simulink model "FCC_replacement"  (R2019b)
settings: Solver=FixedStepDiscrete  StartTime=0.0  StopTime=10.0  FixedStep=0.001  RelTol=1e-3  EnableMultiTasking=on
undefined symbols (not defined in the file or in its folder): DiscIntNeverNeededParam
libraries: simulink x10, HeliLibrary x3
Description:
  | This model represents a flight control system for a helicopter that controls pitch attitude, roll attitude and yaw rate based on pilot inputs from the cyclic and pedals. The flight control computer also closes the loop on three hydrualic actuators and has sensor inputs from three Attitude/Heading Reference Systems.
settings Model: DataDictionary=HeliSystemDD.sldd  sldv_blockreplacement_configurable_lib=FCC_rt_lib  Creator=bpotter  LastModifiedBy=bpotter
settings DataIOCC: LimitDataPoints=on  ReturnWorkspaceOutputs=off
settings OptimizationCC: BlockReduction=off  DefaultParameterBehavior=Inlined  UseDivisionForNetSlopeComputation=on  InitFltsAndDblsToZero=on  EfficientFloat2IntCast=on  EfficientMapNaN2IntZero=off  LifeSpan=inf  MaxStackSize=inf  EfficientTunableParamExpr=on
settings DebuggingCC: SignalInfNanChecking=error  SignalRangeChecking=error  ReadBeforeWriteMsg=EnableAllAsError  WriteAfterWriteMsg=EnableAllAsError  WriteAfterReadMsg=EnableAllAsError  AlgebraicLoopMsg=error  ArtificialAlgebraicLoopMsg=error  SaveWithDisabledLinksMsg=error  SaveWithParameterizedLinksMsg=none  BlockPriorityViolationMsg=error  SolverPrmCheckMsg=error  InheritedTsInSrcMsg=error  SingleTaskRateTransMsg=error  TasksWithSamePriorityMsg=error  SigSpecEnsureSampleTimeMsg=error  CheckMatrixSingularityMsg=error  IntegerOverflowMsg=error  ParameterUnderflowMsg=error  ParameterPrecisionLossMsg=error  ParameterTunabilityLossMsg=error  UnderSpecifiedDataTypeMsg=error  UnnecessaryDatatypeConvMsg=warning  VectorMatrixConversionMsg=error  UnconnectedInputMsg=error  UnconnectedOutputMsg=error  UnconnectedLineMsg=error  SFcnCompatibilityMsg=error  UniqueDataStoreMsg=warning  BusObjectLabelMismatch=error  RootOutportRequireBusObject=error  AssertControl=DisableAll  AllowSymbolicDim=off  ModelReferenceIOMsg=error  ModelReferenceIOMismatchMessage=error  UnknownTsInhSupMsg=error  ModelReferenceDataLoggingMessage=error  StateNameClashWarn=warning  PregeneratedLibrarySubsystemCodeDiagnostic=none  StrictBusMsg=ErrorOnBusTreatedAsVector  NonBusSignalsTreatedAsBus=error  SFInvalidInputDataAccessInChartInitDiag=error  SFTransitionOutsideNaturalParentDiag=error  SFUnreachableExecutionPathDiag=error  SFUndirectedBroadcastEventsDiag=error  SFTransitionActionBeforeConditionDiag=error  SFExecutionAtInitializationDiag=none  IntegerSaturationMsg=error  ArithmeticOperatorsInVariantConditions=warning
settings HardwareCC: ProdBitPerPointer=32  ProdBitPerSizeT=32  ProdBitPerPtrDiffT=32  ProdWordSize=32  ProdHWDeviceType=Intel->x86-32 (Windows32)  TargetIntDivRoundTo=Zero
settings ModelReferenceCC: ModelReferenceNumInstancesAllowed=Single  PropagateSignalLabelsOutOfModel=off
settings SFSimCC: SimUseLocalCustomCode=off  CompileTimeRecursionLimit=0  EnableRuntimeRecursion=off  MATLABDynamicMemAlloc=off  CustomCodeUndefinedFunction=UseInterfaceOnly
settings RTWCC: SystemTargetFile=ert.tlc  TemplateMakefile=ert_default_tmf  GenerateReport=on  RTWUseLocalCustomCode=off  IncludeHyperlinkInReport=on  LaunchReport=on  PortableWordSizes=on  GenerateTraceInfo=on  GenerateTraceReport=on  GenerateTraceReportSl=on  GenerateTraceReportSf=on  GenerateTraceReportEml=on
settings CodeAppCC: ForceParamTrailComments=on  IgnoreCustomStorageClasses=off  MATLABFcnDesc=on  MangleLength=4  StateflowObjectComments=on  ReqsInCode=on
settings ERTTargetCC: TargetLangStandard=C99 (ISO)  UtilityFuncGeneration=Shared location  MultiwordLength=2048  GenerateSampleERTMain=on  IncludeMdlTerminateFcn=off  SuppressErrorStatus=on  SupportAbsoluteTime=off  SupportNonFinite=off  ParenthesesLevel=Maximum  CastingMode=Standards  GenerateSharedConstants=off  ERTCustomFileTemplate=example_file_process.tlc  ERTFilePackagingFormat=Compact  PreserveExpressionOrder=on  PreserveIfCondition=on  ConvertIfToSwitch=off  SuppressUnreachableDefaultCases=off  EnableSignedLeftShifts=off  EnableSignedRightShifts=off
settings ConfigComp: CovMetricSettings=dw  CovHtmlReporting=on  CovSaveCumulativeToWorkspaceVar=on  CovSaveSingleToWorkspaceVar=on  CovExternalEMLEnable=off  CovSFcnEnable=off  DVTestSuiteOptimization=CombinedObjectives (Nonlinear Extended)  DVDetectOutOfBounds=on  DVDesignMinMaxCheck=on  DVRebuildModelRepresentation=Always

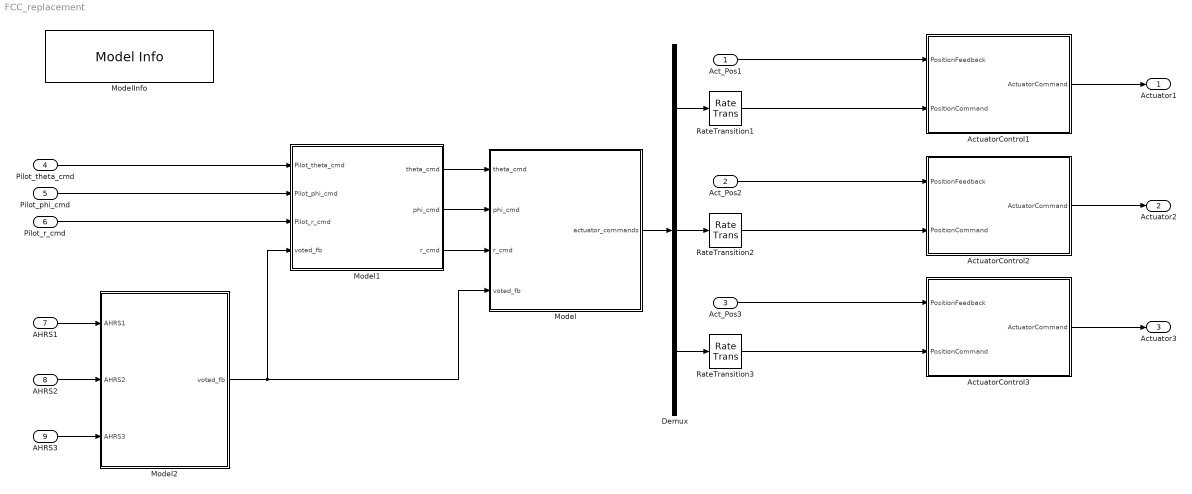
== system FCC_replacement ==
  Act_Pos1 : Inport  RequirementInfo={} %GIDa_bd07c6dd_f370_4b97_930d_e4b4981f6696  OutMin=-32768  OutMax=32767  OutDataTypeStr=int16  PortDimensions=1  SampleTime=0.001
  Act_Pos2 : Inport  RequirementInfo={} %GIDa_befe8f2a_df1a_408c_ad43_982e86d61679  Port=2  OutMin=-32768  OutMax=32767  OutDataTypeStr=int16  PortDimensions=1  SampleTime=0.001
  Act_Pos3 : Inport  RequirementInfo={} %GIDa_31a40888_6c46_41b4_95a0_85353469c339  Port=3  OutMin=-32768  OutMax=32767  OutDataTypeStr=int16  PortDimensions=1  SampleTime=0.001
  Pilot_theta_cmd : Inport  RequirementInfo={} %GIDa_db7610c8_fc0b_436a_9176_d063f912f7d4  Port=4  OutMin=-32768  OutMax=32767  OutDataTypeStr=int16  PortDimensions=1  SampleTime=0.01
  Pilot_phi_cmd : Inport  RequirementInfo={} %GIDa_c88793d4_8072_44c9_b7b8_fa9c7a9d095b  Port=5  OutMin=-32768  OutMax=32767  OutDataTypeStr=int16  PortDimensions=1  SampleTime=0.01
  Pilot_r_cmd : Inport  RequirementInfo={} %GIDa_dcbca35e_d37f_4666_ab6e_90461c32e72b  Port=6  OutMin=-32768  OutMax=32767  OutDataTypeStr=int16  PortDimensions=1  SampleTime=0.01
  AHRS1 : Inport  RequirementInfo={} %GIDa_80750aa2_e003_442f_b031_591405abb5b4  Port=7  OutDataTypeStr=Bus: AHRS_Bus  PortDimensions=1  SampleTime=0.01  BusOutputAsStruct=on
  AHRS2 : Inport  RequirementInfo={} %GIDa_426ecfe9_991d_4f5f_80a1_3ebd9c43cb2d  Port=8  OutDataTypeStr=Bus: AHRS_Bus  PortDimensions=1  SampleTime=0.01  BusOutputAsStruct=on
  AHRS3 : Inport  RequirementInfo={} %GIDa_78c653e8_6a57_498e_82a6_5c1330482b46  Port=9  OutDataTypeStr=Bus: AHRS_Bus  PortDimensions=1  SampleTime=0.01  BusOutputAsStruct=on
  ActuatorControl1 : Subsystem  TreatAsAtomicUnit=on  mask(Sldv ModelReference(Model name:ActuatorLoop) Replacement){ModelName=ActuatorLoop, ParameterArgumentNames=Kp,Kd,Ki, ParameterArgumentValuesAsString=0.00272,2.73,0.339, SimulationMode=Normal, Kd=0.00272, Ki=2.73, Kp=0.339}
      mask help: Replacement for the Model Reference block that references the model ActuatorLoop. If Model arguments are specified on the Model Reference block, then they will appear in the mask parameters.
  ActuatorControl2 : Subsystem  TreatAsAtomicUnit=on  mask(Sldv ModelReference(Model name:ActuatorLoop) Replacement){ModelName=ActuatorLoop, ParameterArgumentNames=Kp,Kd,Ki, ParameterArgumentValuesAsString=0.00272,2.73,0.339, SimulationMode=Normal, Kd=0.00272, Ki=2.73, Kp=0.339}
      mask help: Replacement for the Model Reference block that references the model ActuatorLoop. If Model arguments are specified on the Model Reference block, then they will appear in the mask parameters.
  ActuatorControl3 : Subsystem  TreatAsAtomicUnit=on  mask(Sldv ModelReference(Model name:ActuatorLoop) Replacement){ModelName=ActuatorLoop, ParameterArgumentNames=Kp,Kd,Ki, ParameterArgumentValuesAsString=0.00272,2.73,0.339, SimulationMode=Normal, Kd=0.00272, Ki=2.73, Kp=0.339}
      mask help: Replacement for the Model Reference block that references the model ActuatorLoop. If Model arguments are specified on the Model Reference block, then they will appear in the mask parameters.
  Demux : Demux  Outputs=3
  Model : Subsystem  TreatAsAtomicUnit=on  mask(Sldv ModelReference(Model name:Heli_inner_loop) Replacement){ModelName=Heli_inner_loop, ParameterArgumentNames=, ParameterArgumentValuesAsString=, SimulationMode=Normal}
      mask help: Replacement for the Model Reference block that references the model Heli_inner_loop. If Model arguments are specified on the Model Reference block, then they will appear in the mask parameters.
  Model1 : Subsystem  TreatAsAtomicUnit=on  mask(Sldv ModelReference(Model name:Heli_outer_loop) Replacement){ModelName=Heli_outer_loop, ParameterArgumentNames=, ParameterArgumentValuesAsString=, SimulationMode=Normal}
      mask help: Replacement for the Model Reference block that references the model Heli_outer_loop. If Model arguments are specified on the Model Reference block, then they will appear in the mask parameters.
  Model2 : Subsystem  TreatAsAtomicUnit=on  mask(Sldv ModelReference(Model name:AHRS_voter) Replacement){ModelName=AHRS_voter, ParameterArgumentNames=, ParameterArgumentValuesAsString=, SimulationMode=Normal}
      mask help: Replacement for the Model Reference block that references the model AHRS_voter. If Model arguments are specified on the Model Reference block, then they will appear in the mask parameters.
  ModelInfo : simulink/Model-Wide Utilities/Model Info  Frame=on  DisplayStringWithTags=|  HorizontalTextAlignment=Center  LeftAlignmentValue=0.5
      | Model Name: %<ModelName>
      | Model Version: %<ModelVersion>
      | Last Modified: %<LastModificationDate>
      | 
      | Copyright 2016 The MathWorks, Inc.
  RateTransition1 : RateTransition  OutPortSampleTime=0.001
  RateTransition2 : RateTransition  OutPortSampleTime=0.001
  RateTransition3 : RateTransition  OutPortSampleTime=0.001
  Actuator1 : Outport  RequirementInfo={} %GIDa_0e27a381_736b_4604_a443_1ce3b6bc89bb  VectorParamsAs1DForOutWhenUnconnected=off
  Actuator2 : Outport  RequirementInfo={} %GIDa_ad165c3e_4ab6_4671_aa0b_225d448592bb  Port=2  VectorParamsAs1DForOutWhenUnconnected=off
  Actuator3 : Outport  RequirementInfo={} %GIDa_f2f33165_edb5_46cb_9250_52960ae67539  Port=3  VectorParamsAs1DForOutWhenUnconnected=off
  wires:
  RateTransition1/1 -> ActuatorControl1/2(PositionCommand)
  RateTransition2/1 -> ActuatorControl2/2(PositionCommand)
  RateTransition3/1 -> ActuatorControl3/2(PositionCommand)
  AHRS2/1 -> Model2/2(AHRS2)
  AHRS3/1 -> Model2/3(AHRS3)
  Demux/1 -> RateTransition1/1
  Demux/2 -> RateTransition2/1
  Demux/3 -> RateTransition3/1
  Model/1(actuator_commands) -> Demux/1
  Model1/1(theta_cmd) -> Model/1(theta_cmd)
  Model1/2(phi_cmd) -> Model/2(phi_cmd)
  Model1/3(r_cmd) -> Model/3(r_cmd)
  AHRS1/1 -> Model2/1(AHRS1)
  Pilot_theta_cmd/1 -> Model1/1(Pilot_theta_cmd)
  Pilot_phi_cmd/1 -> Model1/2(Pilot_phi_cmd)
  Pilot_r_cmd/1 -> Model1/3(Pilot_r_cmd)
  Act_Pos1/1 -> ActuatorControl1/1(PositionFeedback)
  Act_Pos2/1 -> ActuatorControl2/1(PositionFeedback)
  Act_Pos3/1 -> ActuatorControl3/1(PositionFeedback)
  ActuatorControl1/1(ActuatorCommand) -> Actuator1/1
  ActuatorControl2/1(ActuatorCommand) -> Actuator2/1
  ActuatorControl3/1(ActuatorCommand) -> Actuator3/1
  Model2/1(voted_fb) -> Model/4(voted_fb), Model1/4(voted_fb)

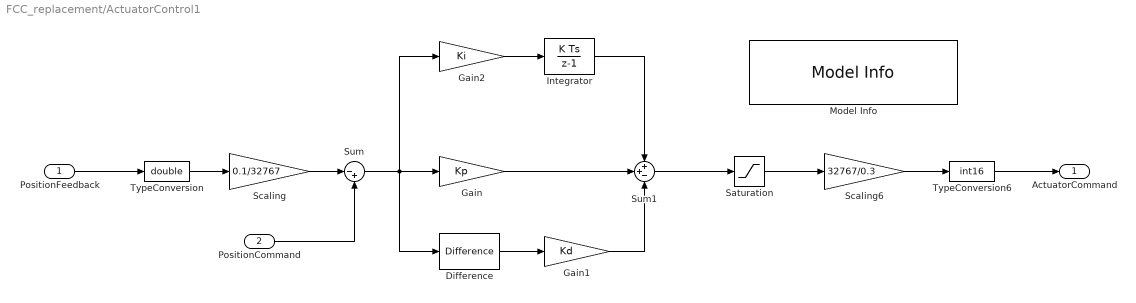
== system FCC_replacement/ActuatorControl1 ==
  PositionFeedback : Inport  OutMin=-32768  OutMax=32767  OutDataTypeStr=int16  PortDimensions=1  SampleTime=[0.001,0]
  PositionCommand : Inport  Port=2  OutMin=-0.1  OutMax=0.1  OutDataTypeStr=double  PortDimensions=1  SampleTime=[0.001,0]
  Difference : simulink/Discrete/Difference  ICPrevInput=0.0  OutMin=[]  OutMax=[]  OutDataType=fixdt(1, 16)  OutScaling=2^-10  DoSatur=off
  Gain : Gain  Gain=Kp
  Gain1 : Gain  Gain=Kd
  Gain2 : Gain  Gain=Ki
  Integrator : DiscreteIntegrator  SampleTime=-1  LimitOutput=on  UpperSaturationLimit=0.1  LowerSaturationLimit=-0.1  ICPrevOutput=DiscIntNeverNeededParam  ICPrevScaledInput=DiscIntNeverNeededParam
      settings: AttributesFormatString="%<LowerSaturationLimit> to  %<UpperSaturationLimit>"
  Model Info : simulink/Model-Wide Utilities/Model Info  Frame=on  DisplayStringWithTags=|  HorizontalTextAlignment=Center  LeftAlignmentValue=0.5
      | Model Name: %<ModelName>
      | Model Version: %<ModelVersion>
      | Last Modified: %<LastModificationDate>
      | 
      | Copyright 2016 The MathWorks, Inc.
  Saturation : Saturate  UpperLimit=0.3  LowerLimit=-0.3
      settings: AttributesFormatString=%<LowerLimit> to %<UpperLimit>
  Scaling : Gain  Gain=0.1/32767
  Scaling6 : Gain  Gain=32767/0.3  SaturateOnIntegerOverflow=on  OutDataTypeStr=Inherit: Same as input
  Sum : Sum  Inputs=|-+
  Sum1 : Sum  Inputs=++-
  TypeConversion : DataTypeConversion  OutDataTypeStr=double
  TypeConversion6 : DataTypeConversion  OutDataTypeStr=int16
  ActuatorCommand : Outport  OutDataTypeStr=int16  PortDimensions=1  SampleTime=[0.001,0]  VectorParamsAs1DForOutWhenUnconnected=off
  wires:
  TypeConversion6/1 -> ActuatorCommand/1
  Saturation/1 -> Scaling6/1
  Scaling6/1 -> TypeConversion6/1
  Scaling/1 -> Sum/1
  TypeConversion/1 -> Scaling/1
  PositionFeedback/1 -> TypeConversion/1
  Gain2/1 -> Integrator/1
  Gain1/1 -> Sum1/3
  Difference/1 -> Gain1/1
  Integrator/1 -> Sum1/1
  Sum1/1 -> Saturation/1
  Gain/1 -> Sum1/2
  Sum/1 -> Difference/1, Gain2/1, Gain/1
  PositionCommand/1 -> Sum/2

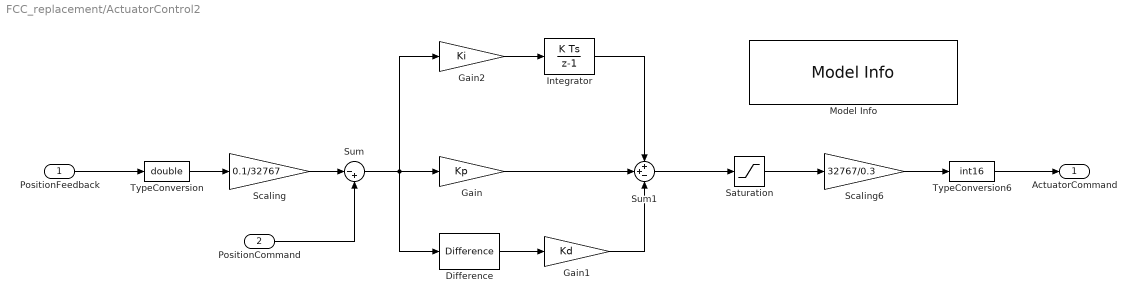
== system FCC_replacement/ActuatorControl2 ==
  PositionFeedback : Inport  OutMin=-32768  OutMax=32767  OutDataTypeStr=int16  PortDimensions=1  SampleTime=[0.001,0]
  PositionCommand : Inport  Port=2  OutMin=-0.1  OutMax=0.1  OutDataTypeStr=double  PortDimensions=1  SampleTime=[0.001,0]
  Difference : simulink/Discrete/Difference  ICPrevInput=0.0  OutMin=[]  OutMax=[]  OutDataType=fixdt(1, 16)  OutScaling=2^-10  DoSatur=off
  Gain : Gain  Gain=Kp
  Gain1 : Gain  Gain=Kd
  Gain2 : Gain  Gain=Ki
  Integrator : DiscreteIntegrator  SampleTime=-1  LimitOutput=on  UpperSaturationLimit=0.1  LowerSaturationLimit=-0.1  ICPrevOutput=DiscIntNeverNeededParam  ICPrevScaledInput=DiscIntNeverNeededParam
      settings: AttributesFormatString="%<LowerSaturationLimit> to  %<UpperSaturationLimit>"
  Model Info : simulink/Model-Wide Utilities/Model Info  Frame=on  DisplayStringWithTags=|  HorizontalTextAlignment=Center  LeftAlignmentValue=0.5
      | Model Name: %<ModelName>
      | Model Version: %<ModelVersion>
      | Last Modified: %<LastModificationDate>
      | 
      | Copyright 2016 The MathWorks, Inc.
  Saturation : Saturate  UpperLimit=0.3  LowerLimit=-0.3
      settings: AttributesFormatString=%<LowerLimit> to %<UpperLimit>
  Scaling : Gain  Gain=0.1/32767
  Scaling6 : Gain  Gain=32767/0.3  SaturateOnIntegerOverflow=on  OutDataTypeStr=Inherit: Same as input
  Sum : Sum  Inputs=|-+
  Sum1 : Sum  Inputs=++-
  TypeConversion : DataTypeConversion  OutDataTypeStr=double
  TypeConversion6 : DataTypeConversion  OutDataTypeStr=int16
  ActuatorCommand : Outport  OutDataTypeStr=int16  PortDimensions=1  SampleTime=[0.001,0]  VectorParamsAs1DForOutWhenUnconnected=off
  wires:
  TypeConversion6/1 -> ActuatorCommand/1
  Saturation/1 -> Scaling6/1
  Scaling6/1 -> TypeConversion6/1
  Scaling/1 -> Sum/1
  TypeConversion/1 -> Scaling/1
  PositionFeedback/1 -> TypeConversion/1
  Gain2/1 -> Integrator/1
  Gain1/1 -> Sum1/3
  Difference/1 -> Gain1/1
  Integrator/1 -> Sum1/1
  Sum1/1 -> Saturation/1
  Gain/1 -> Sum1/2
  Sum/1 -> Difference/1, Gain2/1, Gain/1
  PositionCommand/1 -> Sum/2

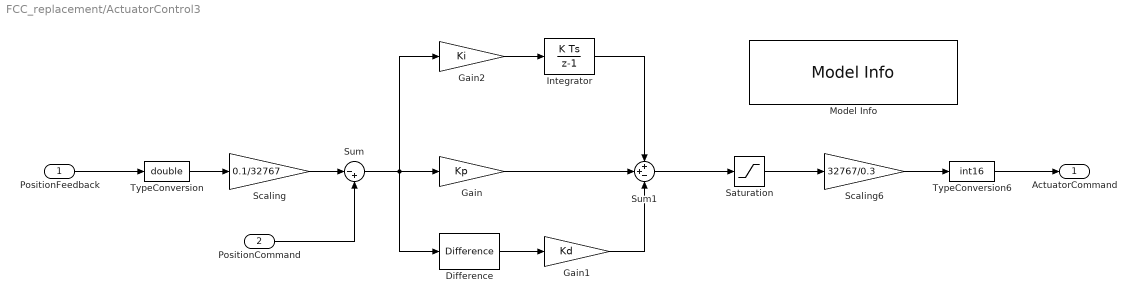
== system FCC_replacement/ActuatorControl3 ==
  PositionFeedback : Inport  OutMin=-32768  OutMax=32767  OutDataTypeStr=int16  PortDimensions=1  SampleTime=[0.001,0]
  PositionCommand : Inport  Port=2  OutMin=-0.1  OutMax=0.1  OutDataTypeStr=double  PortDimensions=1  SampleTime=[0.001,0]
  Difference : simulink/Discrete/Difference  ICPrevInput=0.0  OutMin=[]  OutMax=[]  OutDataType=fixdt(1, 16)  OutScaling=2^-10  DoSatur=off
  Gain : Gain  Gain=Kp
  Gain1 : Gain  Gain=Kd
  Gain2 : Gain  Gain=Ki
  Integrator : DiscreteIntegrator  SampleTime=-1  LimitOutput=on  UpperSaturationLimit=0.1  LowerSaturationLimit=-0.1  ICPrevOutput=DiscIntNeverNeededParam  ICPrevScaledInput=DiscIntNeverNeededParam
      settings: AttributesFormatString="%<LowerSaturationLimit> to  %<UpperSaturationLimit>"
  Model Info : simulink/Model-Wide Utilities/Model Info  Frame=on  DisplayStringWithTags=|  HorizontalTextAlignment=Center  LeftAlignmentValue=0.5
      | Model Name: %<ModelName>
      | Model Version: %<ModelVersion>
      | Last Modified: %<LastModificationDate>
      | 
      | Copyright 2016 The MathWorks, Inc.
  Saturation : Saturate  UpperLimit=0.3  LowerLimit=-0.3
      settings: AttributesFormatString=%<LowerLimit> to %<UpperLimit>
  Scaling : Gain  Gain=0.1/32767
  Scaling6 : Gain  Gain=32767/0.3  SaturateOnIntegerOverflow=on  OutDataTypeStr=Inherit: Same as input
  Sum : Sum  Inputs=|-+
  Sum1 : Sum  Inputs=++-
  TypeConversion : DataTypeConversion  OutDataTypeStr=double
  TypeConversion6 : DataTypeConversion  OutDataTypeStr=int16
  ActuatorCommand : Outport  OutDataTypeStr=int16  PortDimensions=1  SampleTime=[0.001,0]  VectorParamsAs1DForOutWhenUnconnected=off
  wires:
  TypeConversion6/1 -> ActuatorCommand/1
  Saturation/1 -> Scaling6/1
  Scaling6/1 -> TypeConversion6/1
  Scaling/1 -> Sum/1
  TypeConversion/1 -> Scaling/1
  PositionFeedback/1 -> TypeConversion/1
  Gain2/1 -> Integrator/1
  Gain1/1 -> Sum1/3
  Difference/1 -> Gain1/1
  Integrator/1 -> Sum1/1
  Sum1/1 -> Saturation/1
  Gain/1 -> Sum1/2
  Sum/1 -> Difference/1, Gain2/1, Gain/1
  PositionCommand/1 -> Sum/2

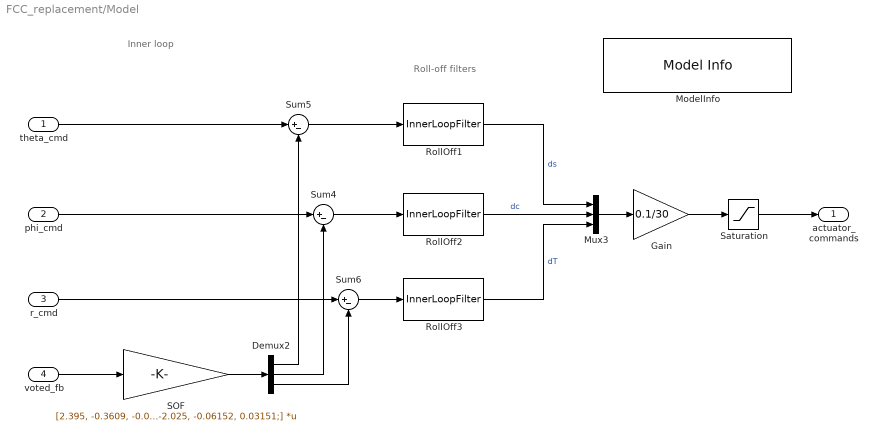
== system FCC_replacement/Model ==
  note: Inner loop
  note: Roll-off filters
  theta_cmd : Inport  OutMin=-30  OutMax=30  OutDataTypeStr=double  PortDimensions=1  SampleTime=[0.01,0]
  phi_cmd : Inport  Port=2  OutMin=-30  OutMax=30  OutDataTypeStr=double  PortDimensions=1  SampleTime=[0.01,0]
  r_cmd : Inport  Port=3  OutMin=-30  OutMax=30  OutDataTypeStr=double  PortDimensions=1  SampleTime=[0.01,0]
  voted_fb : Inport  Port=4  OutMin=-180  OutMax=180  OutDataTypeStr=double  PortDimensions=5  SampleTime=[0.01,0]
  Demux2 : Demux  Outputs=3
  Gain : Gain  Gain=0.1/30
  ModelInfo : simulink/Model-Wide Utilities/Model Info  Frame=on  DisplayStringWithTags=|  HorizontalTextAlignment=Center  LeftAlignmentValue=0.5
      | Model Name: %<ModelName>
      | Model Version: %<ModelVersion>
      | Last Modified: %<LastModificationDate>
      | 
      | Copyright 2016 The MathWorks, Inc.
  Mux3 : Mux  Inputs=3
  RollOff1 : HeliLibrary/InnerLoopFilter  Tag=FilterWizardSubSystem  SystemSampleTime=-1  Latency=0  AutoFrameSizeCalculation=off
      settings: AttributesFormatString=@100Hz
  RollOff2 : HeliLibrary/InnerLoopFilter  Tag=FilterWizardSubSystem  SystemSampleTime=-1  Latency=0  AutoFrameSizeCalculation=off
      settings: AttributesFormatString=@100Hz
  RollOff3 : HeliLibrary/InnerLoopFilter  Tag=FilterWizardSubSystem  SystemSampleTime=-1  Latency=0  AutoFrameSizeCalculation=off
      settings: AttributesFormatString=@100Hz
  SOF : Gain  Gain=[2.395, -0.3609, -0.002145, 0.8087, -0.0205; -0.1427, -1.115, 0.04573, -0.04318, -0.1007; -0.02792, -0.02229, -2.025, -0.06152, 0.03151;]  Multiplication=Matrix(K*u) (u vector)
  Saturation : Saturate  UpperLimit=0.1  LowerLimit=-0.1
  Sum4 : Sum  Inputs=|+-
  Sum5 : Sum  Inputs=|+-
  Sum6 : Sum  Inputs=|+-
  actuator_commands : Outport  OutDataTypeStr=double  PortDimensions=3  SampleTime=[0.01,0]  VectorParamsAs1DForOutWhenUnconnected=off
  wires:
  Saturation/1 -> actuator_commands/1
  Gain/1 -> Saturation/1
  voted_fb/1 -> SOF/1
  Demux2/3 -> Sum6/2
  Demux2/2 -> Sum4/2
  Demux2/1 -> Sum5/2
  Sum6/1 -> RollOff3/1
  r_cmd/1 -> Sum6/1
  phi_cmd/1 -> Sum4/1
  SOF/1 -> Demux2/1
  Sum5/1 -> RollOff1/1
  theta_cmd/1 -> Sum5/1
  RollOff1/1 -> Mux3/1  "ds"
  RollOff2/1 -> Mux3/2  "dc"
  RollOff3/1 -> Mux3/3  "dT"
  Sum4/1 -> RollOff2/1
  Mux3/1 -> Gain/1

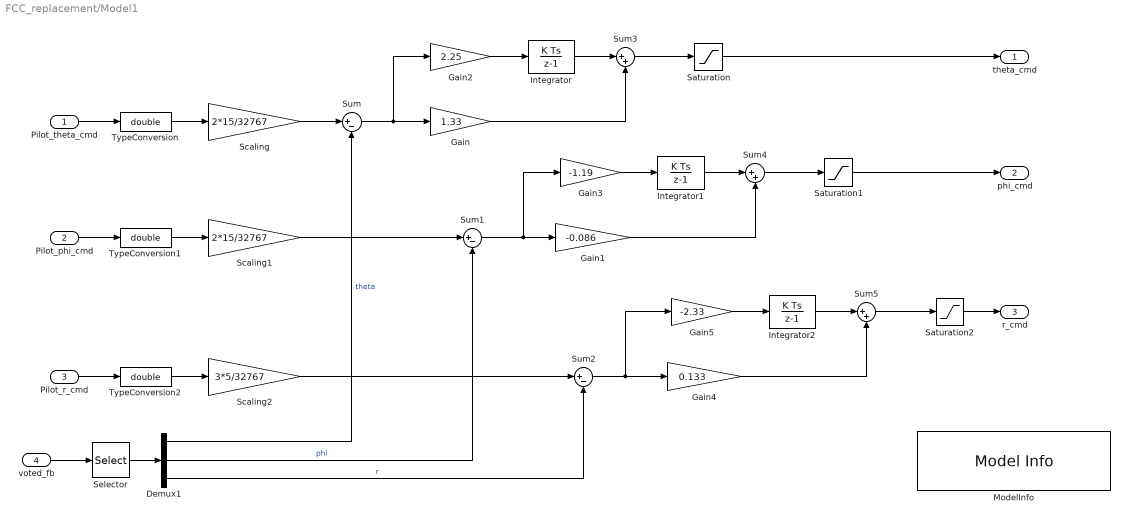
== system FCC_replacement/Model1 ==
  Pilot_theta_cmd : Inport  OutMin=-32768  OutMax=32767  OutDataTypeStr=int16  PortDimensions=1  SampleTime=[0.01,0]
  Pilot_phi_cmd : Inport  Port=2  OutMin=-32768  OutMax=32767  OutDataTypeStr=int16  PortDimensions=1  SampleTime=[0.01,0]
  Pilot_r_cmd : Inport  Port=3  OutMin=-32768  OutMax=32767  OutDataTypeStr=int16  PortDimensions=1  SampleTime=[0.01,0]
  voted_fb : Inport  Port=4  OutMin=-180  OutMax=180  OutDataTypeStr=double  PortDimensions=5  SampleTime=[0.01,0]
  Demux1 : Demux  Outputs=3
  Gain : Gain  Gain=1.33
  Gain1 : Gain  Gain=-0.086
  Gain2 : Gain  Gain=2.25
  Gain3 : Gain  Gain=-1.19
  Gain4 : Gain  Gain=0.133
  Gain5 : Gain  Gain=-2.33
  Integrator : DiscreteIntegrator  SampleTime=-1  LimitOutput=on  UpperSaturationLimit=10  LowerSaturationLimit=-10  ICPrevOutput=DiscIntNeverNeededParam  ICPrevScaledInput=DiscIntNeverNeededParam
      settings: AttributesFormatString="%<LowerSaturationLimit> to  %<UpperSaturationLimit>"
  Integrator1 : DiscreteIntegrator  SampleTime=-1  LimitOutput=on  UpperSaturationLimit=10  LowerSaturationLimit=-10  ICPrevOutput=DiscIntNeverNeededParam  ICPrevScaledInput=DiscIntNeverNeededParam
      settings: AttributesFormatString="%<LowerSaturationLimit> to  %<UpperSaturationLimit>"
  Integrator2 : DiscreteIntegrator  SampleTime=-1  LimitOutput=on  UpperSaturationLimit=10  LowerSaturationLimit=-10  ICPrevOutput=DiscIntNeverNeededParam  ICPrevScaledInput=DiscIntNeverNeededParam
      settings: AttributesFormatString="%<LowerSaturationLimit> to  %<UpperSaturationLimit>"
  ModelInfo : simulink/Model-Wide Utilities/Model Info  Frame=on  DisplayStringWithTags=|  HorizontalTextAlignment=Center  LeftAlignmentValue=0.5
      | Model Name: %<ModelName>
      | Model Version: %<ModelVersion>
      | Last Modified: %<LastModificationDate>
      | 
      | Copyright 2016 The MathWorks, Inc.
  Saturation : Saturate  UpperLimit=30  LowerLimit=-30
      settings: AttributesFormatString=%<LowerLimit> to %<UpperLimit>
  Saturation1 : Saturate  UpperLimit=30  LowerLimit=-30
      settings: AttributesFormatString=%<LowerLimit> to %<UpperLimit>
  Saturation2 : Saturate  UpperLimit=30  LowerLimit=-30
      settings: AttributesFormatString=%<LowerLimit> to %<UpperLimit>
  Scaling : Gain  Gain=2*15/32767
  Scaling1 : Gain  Gain=2*15/32767
  Scaling2 : Gain  Gain=3*5/32767
  Selector : Selector  InputPortWidth=5  IndexOptions=Index vector (dialog)  Indices=[1 2 3]  OutputSizes=1
  Sum : Sum  Inputs=|+-  InputSameDT=on  OutDataTypeStr=Inherit: Same as first input
  Sum1 : Sum  Inputs=|+-  InputSameDT=on  OutDataTypeStr=Inherit: Same as first input
  Sum2 : Sum  Inputs=|+-  InputSameDT=on  OutDataTypeStr=Inherit: Same as first input
  Sum3 : Sum  Inputs=|++
  Sum4 : Sum  Inputs=|++
  Sum5 : Sum  Inputs=|++
  TypeConversion : DataTypeConversion  OutDataTypeStr=double
  TypeConversion1 : DataTypeConversion  OutDataTypeStr=double
  TypeConversion2 : DataTypeConversion  OutDataTypeStr=double
  theta_cmd : Outport  OutDataTypeStr=double  PortDimensions=1  SampleTime=[0.01,0]  VectorParamsAs1DForOutWhenUnconnected=off
  phi_cmd : Outport  Port=2  OutDataTypeStr=double  PortDimensions=1  SampleTime=[0.01,0]  VectorParamsAs1DForOutWhenUnconnected=off
  r_cmd : Outport  Port=3  OutDataTypeStr=double  PortDimensions=1  SampleTime=[0.01,0]  VectorParamsAs1DForOutWhenUnconnected=off
  wires:
  Scaling2/1 -> Sum2/1
  Pilot_r_cmd/1 -> TypeConversion2/1
  Scaling1/1 -> Sum1/1
  Pilot_phi_cmd/1 -> TypeConversion1/1
  Scaling/1 -> Sum/1
  Pilot_theta_cmd/1 -> TypeConversion/1
  TypeConversion/1 -> Scaling/1
  TypeConversion1/1 -> Scaling1/1
  TypeConversion2/1 -> Scaling2/1
  Saturation2/1 -> r_cmd/1
  Sum2/1 -> Gain5/1, Gain4/1
  Gain5/1 -> Integrator2/1
  Integrator2/1 -> Sum5/1
  Sum5/1 -> Saturation2/1
  Gain4/1 -> Sum5/2
  Saturation1/1 -> phi_cmd/1
  Gain3/1 -> Integrator1/1
  Integrator1/1 -> Sum4/1
  Sum4/1 -> Saturation1/1
  Gain1/1 -> Sum4/2
  Sum1/1 -> Gain3/1, Gain1/1
  Saturation/1 -> theta_cmd/1
  Gain2/1 -> Integrator/1
  Integrator/1 -> Sum3/1
  Sum3/1 -> Saturation/1
  Gain/1 -> Sum3/2
  Sum/1 -> Gain/1, Gain2/1
  voted_fb/1 -> Selector/1
  Demux1/3 -> Sum2/2  "r"
  Demux1/2 -> Sum1/2  "phi"
  Demux1/1 -> Sum/2  "theta"
  Selector/1 -> Demux1/1

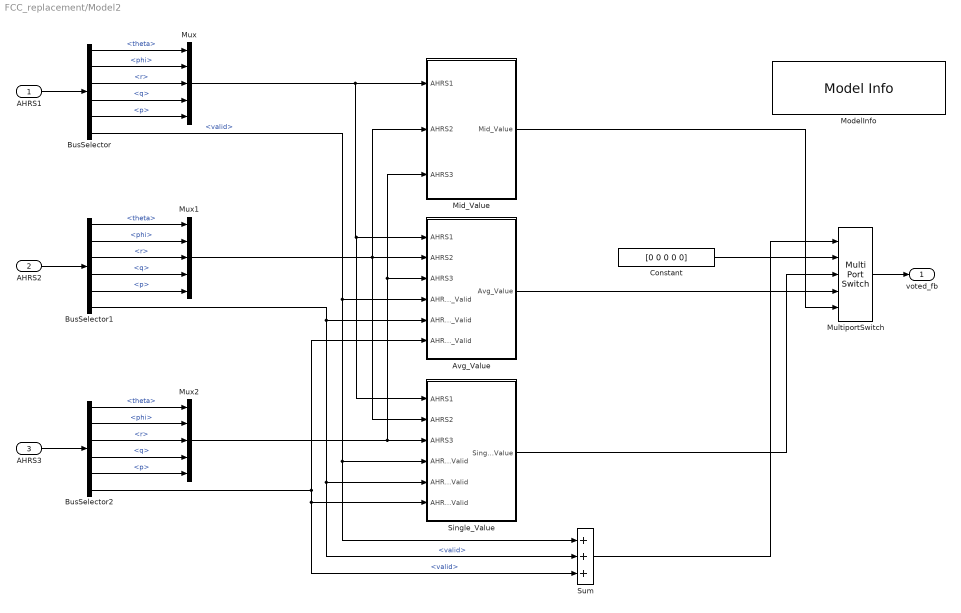
== system FCC_replacement/Model2 ==
  AHRS1 : Inport  OutDataTypeStr=Bus: AHRS_Bus  PortDimensions=1  SampleTime=[0.01,0]  BusOutputAsStruct=on
  AHRS2 : Inport  Port=2  OutDataTypeStr=Bus: AHRS_Bus  PortDimensions=1  SampleTime=[0.01,0]  BusOutputAsStruct=on
  AHRS3 : Inport  Port=3  OutDataTypeStr=Bus: AHRS_Bus  PortDimensions=1  SampleTime=[0.01,0]  BusOutputAsStruct=on
  Avg_Value : Subsystem  TreatAsAtomicUnit=on  RTWFcnName=Avg_Value
      settings: RTWSystemCode=Inline  RTWFcnNameOpts=User specified
  BusSelector : BusSelector  OutputSignals=theta,phi,r,q,p,valid
  BusSelector1 : BusSelector  OutputSignals=theta,phi,r,q,p,valid
  BusSelector2 : BusSelector  OutputSignals=theta,phi,r,q,p,valid
  Constant : Constant  Value=[0 0 0 0 0]
  Mid_Value : Subsystem  TreatAsAtomicUnit=on  RTWFcnName=Mid_Value
      settings: RTWSystemCode=Inline  RTWFcnNameOpts=User specified
  ModelInfo : simulink/Model-Wide Utilities/Model Info  Frame=on  DisplayStringWithTags=|  HorizontalTextAlignment=Center  LeftAlignmentValue=0.5
      | Model Name: %<ModelName>
      | Model Version: %<ModelVersion>
      | Last Modified: %<LastModificationDate>
      | 
      | Copyright 2016 The MathWorks, Inc.
  MultiportSwitch : MultiPortSwitch  DataPortOrder=Zero-based contiguous  Inputs=4  DiagnosticForDefault=None  zeroidx=on
  Mux : Mux  Inputs=5
  Mux1 : Mux  Inputs=5
  Mux2 : Mux  Inputs=5
  Single_Value : Subsystem  TreatAsAtomicUnit=on  RTWFcnName=Single_Value
      settings: RTWSystemCode=Inline  RTWFcnNameOpts=User specified
  Sum : Sum  Inputs=+++  OutDataTypeStr=uint32
  voted_fb : Outport  OutDataTypeStr=double  PortDimensions=5  SampleTime=[0.01,0]  VectorParamsAs1DForOutWhenUnconnected=off
  wires:
  BusSelector2/6 -> Single_Value/6(AHRS3_Valid), Sum/3, Avg_Value/6(AHRS3_Valid)  "<valid>"
  BusSelector2/5 -> Mux2/5  "<p>"
  BusSelector2/4 -> Mux2/4  "<q>"
  BusSelector2/3 -> Mux2/3  "<r>"
  BusSelector2/2 -> Mux2/2  "<phi>"
  BusSelector2/1 -> Mux2/1  "<theta>"
  AHRS3/1 -> BusSelector2/1
  Mux2/1 -> Mid_Value/3(AHRS3), Avg_Value/3(AHRS3), Single_Value/3(AHRS3)
  BusSelector1/6 -> Avg_Value/5(AHRS2_Valid), Sum/2, Single_Value/5(AHRS2_Valid)  "<valid>"
  Mux1/1 -> Single_Value/2(AHRS2), Mid_Value/2(AHRS2), Avg_Value/2(AHRS2)
  AHRS2/1 -> BusSelector1/1
  BusSelector1/1 -> Mux1/1  "<theta>"
  BusSelector1/2 -> Mux1/2  "<phi>"
  BusSelector1/3 -> Mux1/3  "<r>"
  BusSelector1/4 -> Mux1/4  "<q>"
  BusSelector1/5 -> Mux1/5  "<p>"
  Mux/1 -> Single_Value/1(AHRS1), Avg_Value/1(AHRS1), Mid_Value/1(AHRS1)
  BusSelector/5 -> Mux/5  "<p>"
  BusSelector/4 -> Mux/4  "<q>"
  BusSelector/3 -> Mux/3  "<r>"
  BusSelector/2 -> Mux/2  "<phi>"
  BusSelector/1 -> Mux/1  "<theta>"
  BusSelector/6 -> Single_Value/4(AHRS1_Valid), Sum/1, Avg_Value/4(AHRS1_Valid)  "<valid>"
  AHRS1/1 -> BusSelector/1
  Constant/1 -> MultiportSwitch/2
  Single_Value/1(Single_Value) -> MultiportSwitch/3
  Avg_Value/1(Avg_Value) -> MultiportSwitch/4
  Mid_Value/1(Mid_Value) -> MultiportSwitch/5
  Sum/1 -> MultiportSwitch/1
  MultiportSwitch/1 -> voted_fb/1

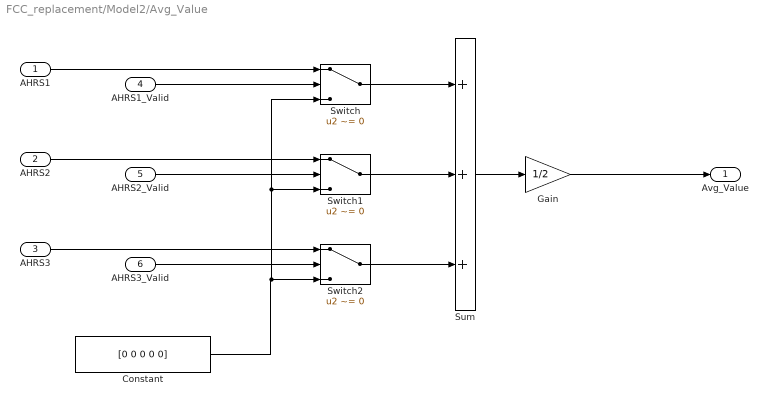
== system FCC_replacement/Model2/Avg_Value ==
  AHRS1 : Inport
  AHRS2 : Inport  Port=2
  AHRS3 : Inport  Port=3
  AHRS1_Valid : Inport  Port=4  OutDataTypeStr=boolean  PortDimensions=1
  AHRS2_Valid : Inport  Port=5  OutDataTypeStr=boolean  PortDimensions=1
  AHRS3_Valid : Inport  Port=6  OutDataTypeStr=boolean  PortDimensions=1
  Constant : Constant  Value=[0 0 0 0 0]
  Gain : Gain  Gain=1/2
  Sum : Sum  Inputs=+++
  Switch : Switch  Criteria=u2 ~= 0
  Switch1 : Switch  Criteria=u2 ~= 0
  Switch2 : Switch  Criteria=u2 ~= 0
  Avg_Value : Outport  VectorParamsAs1DForOutWhenUnconnected=off
  wires:
  Gain/1 -> Avg_Value/1
  Sum/1 -> Gain/1
  AHRS1_Valid/1 -> Switch/2
  AHRS1/1 -> Switch/1
  Switch/1 -> Sum/1
  Switch1/1 -> Sum/2
  Switch2/1 -> Sum/3
  AHRS2_Valid/1 -> Switch1/2
  AHRS3_Valid/1 -> Switch2/2
  AHRS2/1 -> Switch1/1
  AHRS3/1 -> Switch2/1
  Constant/1 -> Switch/3, Switch1/3, Switch2/3

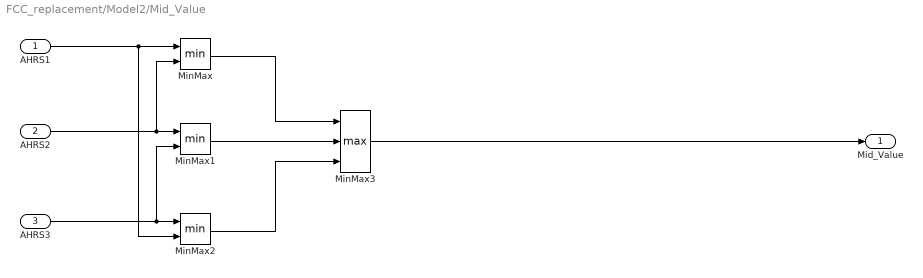
== system FCC_replacement/Model2/Mid_Value ==
  AHRS1 : Inport
  AHRS2 : Inport  Port=2
  AHRS3 : Inport  Port=3
  MinMax : MinMax  Inputs=2
  MinMax1 : MinMax  Inputs=2
  MinMax2 : MinMax  Inputs=2
  MinMax3 : MinMax  Function=max  Inputs=3
  Mid_Value : Outport  VectorParamsAs1DForOutWhenUnconnected=off
  wires:
  AHRS1/1 -> MinMax2/2, MinMax/1
  AHRS3/1 -> MinMax1/2, MinMax2/1
  AHRS2/1 -> MinMax/2, MinMax1/1
  MinMax1/1 -> MinMax3/2
  MinMax/1 -> MinMax3/1
  MinMax2/1 -> MinMax3/3
  MinMax3/1 -> Mid_Value/1

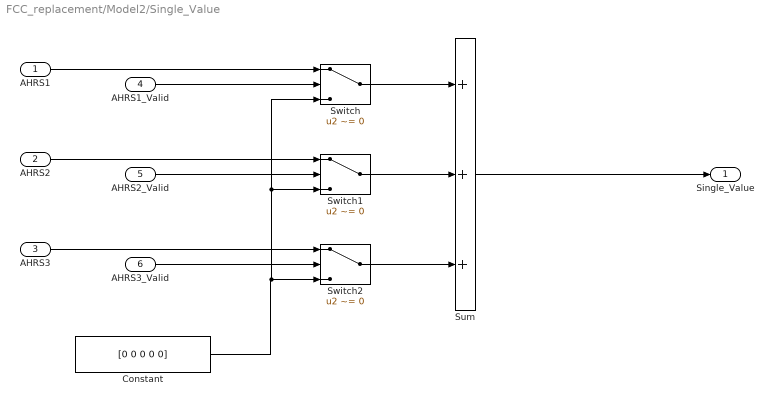
== system FCC_replacement/Model2/Single_Value ==
  AHRS1 : Inport
  AHRS2 : Inport  Port=2
  AHRS3 : Inport  Port=3
  AHRS1_Valid : Inport  Port=4  OutDataTypeStr=boolean  PortDimensions=1
  AHRS2_Valid : Inport  Port=5  OutDataTypeStr=boolean  PortDimensions=1
  AHRS3_Valid : Inport  Port=6  OutDataTypeStr=boolean  PortDimensions=1
  Constant : Constant  Value=[0 0 0 0 0]
  Sum : Sum  Inputs=+++
  Switch : Switch  Criteria=u2 ~= 0
  Switch1 : Switch  Criteria=u2 ~= 0
  Switch2 : Switch  Criteria=u2 ~= 0
  Single_Value : Outport  VectorParamsAs1DForOutWhenUnconnected=off
  wires:
  Constant/1 -> Switch2/3, Switch1/3, Switch/3
  AHRS3/1 -> Switch2/1
  AHRS2/1 -> Switch1/1
  AHRS3_Valid/1 -> Switch2/2
  AHRS2_Valid/1 -> Switch1/2
  Switch2/1 -> Sum/3
  Switch1/1 -> Sum/2
  Switch/1 -> Sum/1
  AHRS1/1 -> Switch/1
  AHRS1_Valid/1 -> Switch/2
  Sum/1 -> Single_Value/1
